simulink model "cell_ecm_2rc"  (R2024b)
settings: Solver=ode4  StartTime=0.0  StopTime=T_stop  FixedStep=0.1  RelTol=1e-3
undefined symbols (not defined in the file): C1_data, C2_data, cp_cell, h_amb, h_cool, m_cell, OCV_data, R0_data, R1_data, R2_data, SoC_bp_ecm, SoC_bp_ocv, T_bp
settings Model: Creator=rayen  LastModifiedBy=rayen
settings OptimizationCC: ZeroExternalMemoryAtStartup=off  ZeroInternalMemoryAtStartup=off
settings DebuggingCC: AlgebraicLoopMsg=error
settings SFSimCC: SimTargetLang=C++
settings RTWCC: TargetLang=C++
settings GRTTargetCC: TargetLangStandard=C++11 (ISO)  CodeInterfacePackaging=C++ class

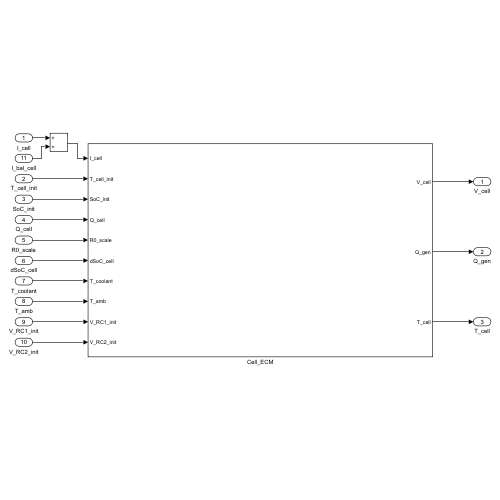
[thumbnail: Simulink's stored preview of the top-level diagram]
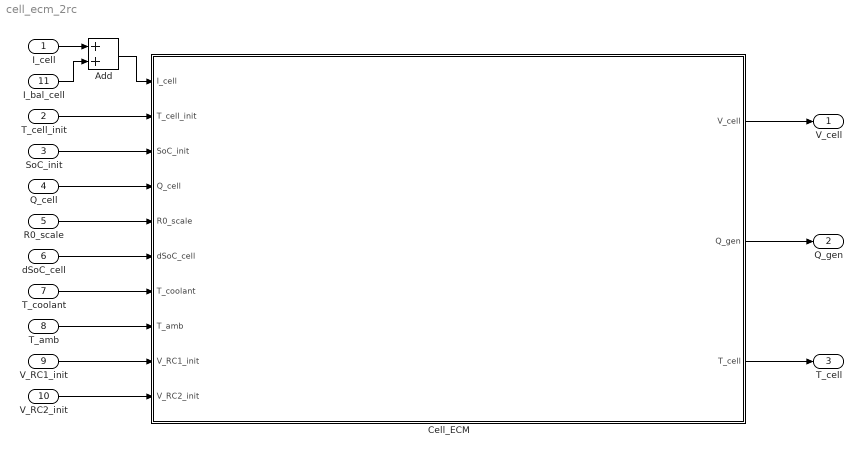
== system cell_ecm_2rc ==
  I_cell : Inport  OutDataTypeStr=double
  T_cell_init : Inport  Port=2  OutDataTypeStr=double
  SoC_init : Inport  Port=3  OutDataTypeStr=double
  Q_cell : Inport  Port=4  OutDataTypeStr=double
  R0_scale : Inport  Port=5  OutDataTypeStr=double
  dSoC_cell : Inport  Port=6  OutDataTypeStr=double
  T_coolant : Inport  Port=7  OutDataTypeStr=double
  T_amb : Inport  Port=8  OutDataTypeStr=double
  V_RC1_init : Inport  Port=9  OutDataTypeStr=double
  V_RC2_init : Inport  Port=10  OutDataTypeStr=double
  I_bal_cell : Inport  Port=11  OutDataTypeStr=double
  Add : Sum
  Cell_ECM : Subsystem
  V_cell : Outport  OutDataTypeStr=double
  Q_gen : Outport  Port=2  OutDataTypeStr=double
  T_cell : Outport  Port=3  OutDataTypeStr=double
  wires:
  Cell_ECM/2(Q_gen) -> Q_gen/1
  Cell_ECM/3(T_cell) -> T_cell/1
  I_cell/1 -> Add/1
  T_cell_init/1 -> Cell_ECM/2(T_cell_init)
  SoC_init/1 -> Cell_ECM/3(SoC_init)
  Q_cell/1 -> Cell_ECM/4(Q_cell)
  R0_scale/1 -> Cell_ECM/5(R0_scale)
  T_coolant/1 -> Cell_ECM/7(T_coolant)
  dSoC_cell/1 -> Cell_ECM/6(dSoC_cell)
  T_amb/1 -> Cell_ECM/8(T_amb)
  Cell_ECM/1(V_cell) -> V_cell/1
  V_RC1_init/1 -> Cell_ECM/9(V_RC1_init)
  V_RC2_init/1 -> Cell_ECM/10(V_RC2_init)
  Add/1 -> Cell_ECM/1(I_cell)
  I_bal_cell/1 -> Add/2

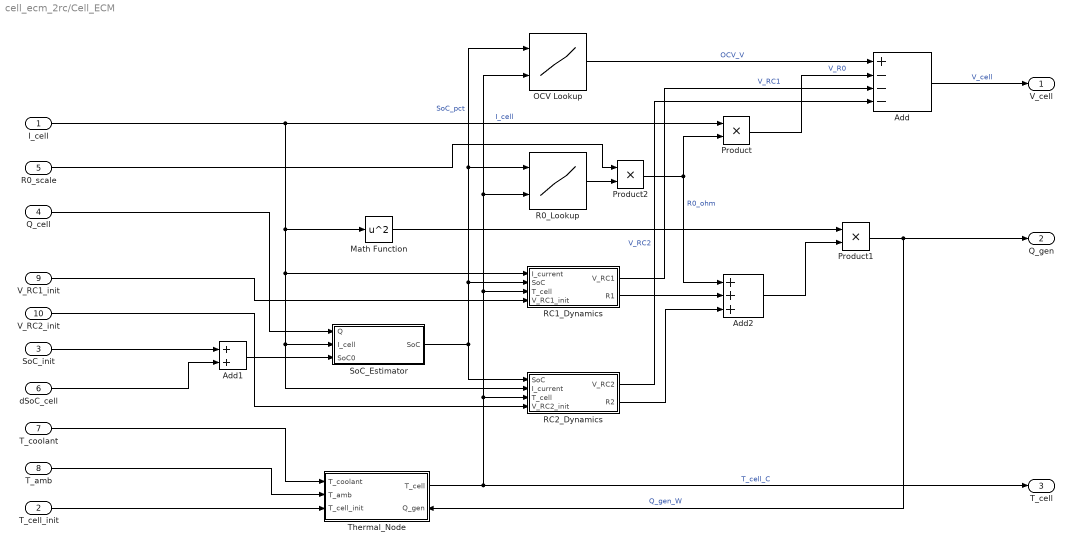
== system cell_ecm_2rc/Cell_ECM ==
  I_cell : Inport  OutDataTypeStr=double
  T_cell_init : Inport  Port=2  OutDataTypeStr=double
  SoC_init : Inport  Port=3  OutDataTypeStr=double
  Q_cell : Inport  Port=4  OutDataTypeStr=double
  R0_scale : Inport  Port=5  OutDataTypeStr=double
  dSoC_cell : Inport  Port=6  OutDataTypeStr=double
  T_coolant : Inport  Port=7  OutDataTypeStr=double
  T_amb : Inport  Port=8  OutDataTypeStr=double
  V_RC1_init : Inport  Port=9  OutDataTypeStr=double
  V_RC2_init : Inport  Port=10  OutDataTypeStr=double
  Add : Sum  Inputs=+---
  Add1 : Sum
  Add2 : Sum  Inputs=+++
  Math Function : Math  Operator=square
  OCV Lookup : Lookup_n-D  BreakpointsForDimension1=SoC_bp_ocv  BreakpointsForDimension2=T_bp  Table=OCV_data  ExtrapMethod=Clip  InternalRulePriority=Speed  RndMeth=Simplest
      settings: InputPortMap=u0,u1
  Product : Product
  Product1 : Product
  Product2 : Product
  R0_Lookup : Lookup_n-D  BreakpointsForDimension1=SoC_bp_ecm  BreakpointsForDimension2=T_bp  Table=R0_data  ExtrapMethod=Clip  InternalRulePriority=Speed  RndMeth=Simplest
      settings: InputPortMap=u0,u1
  RC1_Dynamics : Subsystem
  RC2_Dynamics : Subsystem
  SoC_Estimator : Subsystem
  Thermal_Node : Subsystem
      settings: PortSchema="{\"entries\":[{\"content\":{\"sides\":[{\"content\":{\"connectorIds\":[\"In1\",\"In2\",\"In3\"]},\"type\":\"ConnectorPlacement.EquallySpacedRectSide\",\"uuid\":\"330ff2b2-ad4a-4cd6-be2c-08a04cf77092\"},{\"content\":{\"connectorIds\":[\"Out1\",\"In4\"],\"side\":\"RIGHT\"},\"type\":\"ConnectorPlacement.EquallySpacedRectSide\",\"uuid\":\"26baba41-460a-4ab6-b49f-57d996f6b809\"},{\"content\":{\"side\":\"TOP\"},\"type\":\"ConnectorPlacement.EquallySpacedRectSide\",\"uuid\":\"b66dd53e-2dd2-4f10-a69c-b4301f9f0c58\"}]},\"type\":\"ConnectorPlacement.EquallySpacedConnector\",\"uuid\":\"1cdda253-128a-4431-b557-2556e8c7cf9c\"}],\"packageUris\":[\"http://schema.mathworks.com/mf0/Connector/R2020b\"],\"version\":\"1.0\"}"
  V_cell : Outport  OutDataTypeStr=double
  Q_gen : Outport  Port=2  OutDataTypeStr=double
  T_cell : Outport  Port=3  OutDataTypeStr=double
  wires:
  I_cell/1 -> Math Function/1, RC2_Dynamics/2(I_current), SoC_Estimator/2(I_cell), RC1_Dynamics/1(I_current), Product/1  "I_cell"
  RC1_Dynamics/1(V_RC1) -> Add/3  "V_RC1"
  OCV Lookup/1 -> Add/1  "OCV_V"
  Add/1 -> V_cell/1  "V_cell"
  SoC_Estimator/1(SoC) -> OCV Lookup/1, R0_Lookup/1, RC1_Dynamics/2(SoC), RC2_Dynamics/1(SoC)  "SoC_pct"
  RC2_Dynamics/1(V_RC2) -> Add/4  "V_RC2"
  Product/1 -> Add/2  "V_R0"
  SoC_init/1 -> Add1/1
  Add1/1 -> SoC_Estimator/3(SoC0)
  R0_Lookup/1 -> Product2/2
  Product2/1 -> Add2/1, Product/2  "R0_ohm"
  dSoC_cell/1 -> Add1/2
  R0_scale/1 -> Product2/1
  Q_cell/1 -> SoC_Estimator/1(Q)
  T_coolant/1 -> Thermal_Node/1(T_coolant)
  T_amb/1 -> Thermal_Node/2(T_amb)
  T_cell_init/1 -> Thermal_Node/3(T_cell_init)
  Thermal_Node/1(T_cell) -> RC2_Dynamics/3(T_cell), R0_Lookup/2, OCV Lookup/2, RC1_Dynamics/3(T_cell), T_cell/1  "T_cell_C"
  RC1_Dynamics/2(R1) -> Add2/2
  RC2_Dynamics/2(R2) -> Add2/3
  Add2/1 -> Product1/2
  Math Function/1 -> Product1/1
  Product1/1 -> Thermal_Node/4(Q_gen), Q_gen/1  "Q_gen_W"
  V_RC1_init/1 -> RC1_Dynamics/4(V_RC1_init)
  V_RC2_init/1 -> RC2_Dynamics/4(V_RC2_init)

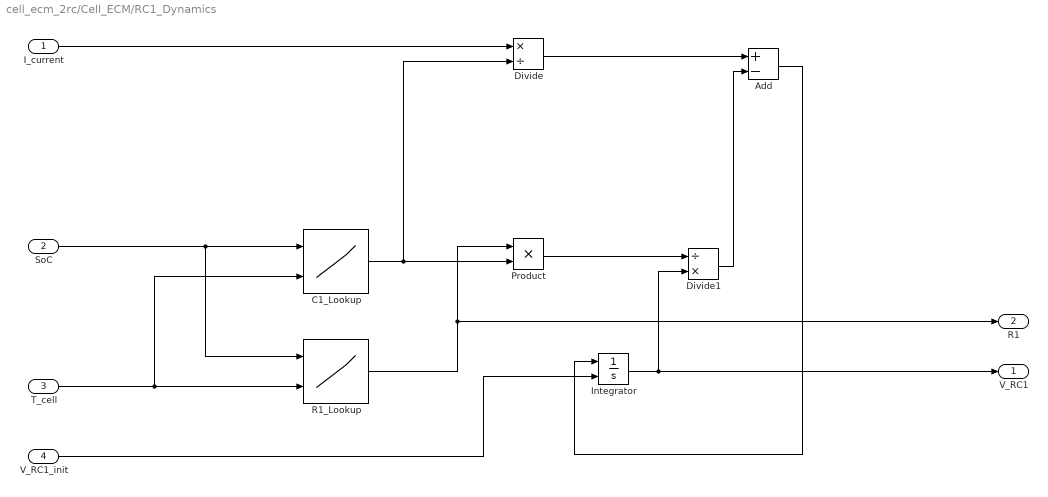
== system cell_ecm_2rc/Cell_ECM/RC1_Dynamics ==
  I_current : Inport
  SoC : Inport  Port=2
  T_cell : Inport  Port=3
  V_RC1_init : Inport  Port=4
  Add : Sum  Inputs=+-
  C1_Lookup : Lookup_n-D  BreakpointsForDimension1=SoC_bp_ecm  BreakpointsForDimension2=T_bp  Table=C1_data  ExtrapMethod=Clip  InternalRulePriority=Speed  RndMeth=Simplest
      settings: InputPortMap=u0,u1
  Divide : Product  Inputs=*/
  Divide1 : Product  Inputs=/*
  Integrator : Integrator  InitialConditionSource=external
  Product : Product
  R1_Lookup : Lookup_n-D  BreakpointsForDimension1=SoC_bp_ecm  BreakpointsForDimension2=T_bp  Table=R1_data  ExtrapMethod=Clip  InternalRulePriority=Speed  RndMeth=Simplest
      settings: InputPortMap=u0,u1
  V_RC1 : Outport
  R1 : Outport  Port=2
  wires:
  Divide/1 -> Add/1
  C1_Lookup/1 -> Divide/2, Product/2
  Add/1 -> Integrator/1
  Divide1/1 -> Add/2
  Product/1 -> Divide1/1
  Integrator/1 -> Divide1/2, V_RC1/1
  R1_Lookup/1 -> Product/1, R1/1
  SoC/1 -> R1_Lookup/1, C1_Lookup/1
  T_cell/1 -> C1_Lookup/2, R1_Lookup/2
  I_current/1 -> Divide/1
  V_RC1_init/1 -> Integrator/2

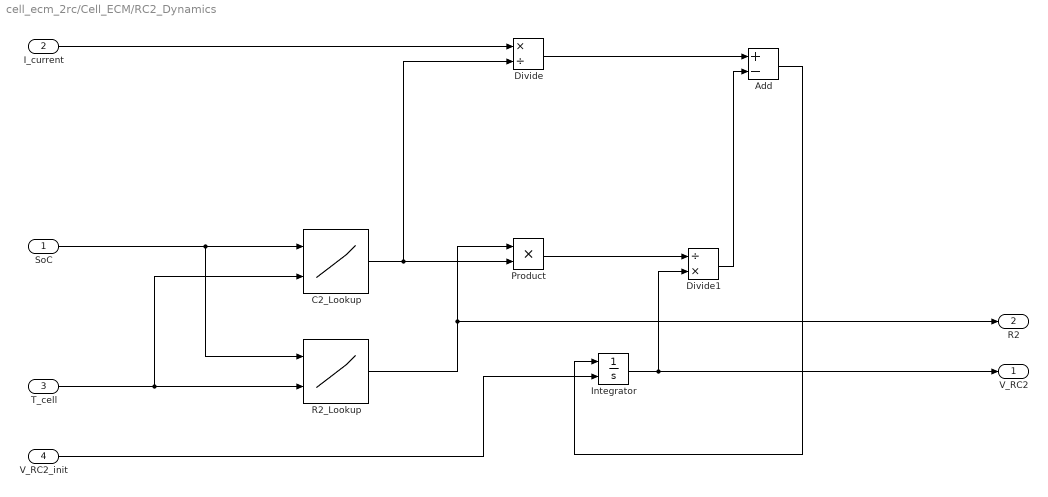
== system cell_ecm_2rc/Cell_ECM/RC2_Dynamics ==
  SoC : Inport
  I_current : Inport  Port=2
  T_cell : Inport  Port=3
  V_RC2_init : Inport  Port=4
  Add : Sum  Inputs=+-
  C2_Lookup : Lookup_n-D  BreakpointsForDimension1=SoC_bp_ecm  BreakpointsForDimension2=T_bp  Table=C2_data  ExtrapMethod=Clip  InternalRulePriority=Speed  RndMeth=Simplest
      settings: InputPortMap=u0,u1
  Divide : Product  Inputs=*/
  Divide1 : Product  Inputs=/*
  Integrator : Integrator  InitialConditionSource=external
  Product : Product
  R2_Lookup : Lookup_n-D  BreakpointsForDimension1=SoC_bp_ecm  BreakpointsForDimension2=T_bp  Table=R2_data  ExtrapMethod=Clip  InternalRulePriority=Speed  RndMeth=Simplest
      settings: InputPortMap=u0,u1
  V_RC2 : Outport
  R2 : Outport  Port=2
  wires:
  I_current/1 -> Divide/1
  Product/1 -> Divide1/1
  C2_Lookup/1 -> Divide/2, Product/2
  T_cell/1 -> R2_Lookup/2, C2_Lookup/2
  Integrator/1 -> Divide1/2, V_RC2/1
  SoC/1 -> R2_Lookup/1, C2_Lookup/1
  Add/1 -> Integrator/1
  Divide1/1 -> Add/2
  Divide/1 -> Add/1
  R2_Lookup/1 -> R2/1, Product/1
  V_RC2_init/1 -> Integrator/2

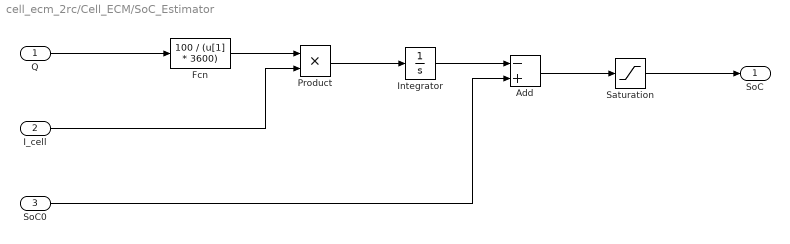
== system cell_ecm_2rc/Cell_ECM/SoC_Estimator ==
  Q : Inport
  I_cell : Inport  Port=2
  SoC0 : Inport  Port=3
  Add : Sum  Inputs=-+
  Fcn : Fcn  Expr=100 / (u[1] * 3600)
  Integrator : Integrator  UpperSaturationLimit=200  LowerSaturationLimit=-200
  Product : Product
  Saturation : Saturate  UpperLimit=100  LowerLimit=0
  SoC : Outport
  wires:
  Saturation/1 -> SoC/1
  Q/1 -> Fcn/1
  I_cell/1 -> Product/2
  Fcn/1 -> Product/1
  Product/1 -> Integrator/1
  Integrator/1 -> Add/1
  SoC0/1 -> Add/2
  Add/1 -> Saturation/1

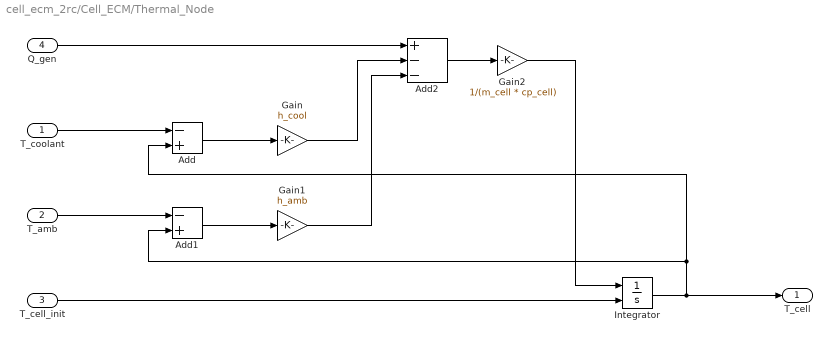
== system cell_ecm_2rc/Cell_ECM/Thermal_Node ==
  T_coolant : Inport
  T_amb : Inport  Port=2
  T_cell_init : Inport  Port=3
  Q_gen : Inport  Port=4
  Add : Sum  Inputs=-+
  Add1 : Sum  Inputs=-+
  Add2 : Sum  Inputs=+--
  Gain : Gain  Gain=h_cool
  Gain1 : Gain  Gain=h_amb
  Gain2 : Gain  Gain=1/(m_cell * cp_cell)
  Integrator : Integrator  InitialConditionSource=external
  T_cell : Outport
  wires:
  T_cell_init/1 -> Integrator/2
  Integrator/1 -> Add1/2, Add/2, T_cell/1
  T_coolant/1 -> Add/1
  Add/1 -> Gain/1
  T_amb/1 -> Add1/1
  Add1/1 -> Gain1/1
  Q_gen/1 -> Add2/1
  Gain/1 -> Add2/2
  Gain1/1 -> Add2/3
  Gain2/1 -> Integrator/1
  Add2/1 -> Gain2/1
